simulink model "Events4"  (Simulink 5.0)
settings: Solver=ode45  StartTime=0.0  StopTime=10.0  RelTol=1e-3
settings Model: Creator=scaife  LastModifiedBy=scaife  ExtModeAutoUpdateStatusClock=off

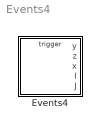
== system Events4 ==
  Events4 : Stateflow chart

== stateflow chart Events4 ==
  state TOP
    state A [parallel]
      state A1/
        en:y++;
        ex:y--;
      state A2/
        en:y+=10;
        ex:y-=10;
      (default) -> A1
      A1 -> A2 : E/I;z++;
      A2 -> A1 : E/J;
          | z+=100;
    state B [parallel]
      state B1
        state B1a/
          en:E;x++;
        state B1b/
          en:E;x++;
        B1a -> B1b : G
        B1b -> B1a : G
        (default) -> B1a
      state B2
        state B2a
        state B2b
        B2a -> B2b : F/E;
            | x++;
        B2b -> B2a : F/E;
            | x++;
        (default) -> B2a
      (default) -> B1
      B1 -> B2 : H
      B2 -> B1 : H
  (default) -> TOP
  data: y output int32; z output int32; x output int32
  events: F input RISING_EDGE_EVENT; G input RISING_EDGE_EVENT; H input RISING_EDGE_EVENT; E local EITHER_EDGE_EVENT; I output FUNCTION_CALL_EVENT; J output FUNCTION_CALL_EVENT
